simulink library "Ice_Storage"  (R2018b)
settings: Solver=ode45  StartTime=0.0  StopTime=10.0  RelTol=1e-3  EnableMultiTasking=on
undefined symbols (not defined in the file): A_earth, delta_grd, h_ini, U_earth, UA_tank, V_earth, ztilde
libraries: carnot x2
settings Model: Creator=drhf  LastModifiedBy=drhf
settings DataIOCC: LimitDataPoints=on  SaveFormat=Array  SignalLoggingSaveFormat=ModelDataLogs
settings OptimizationCC: ExpressionDepthLimit=2147483647  LifeSpan=inf
settings DebuggingCC: UnderspecifiedInitializationDetection=Classic  MergeDetectMultiDrivingBlocksExec=none  SolverPrmCheckMsg=warning  FcnCallInpInsideContextMsg=warning  StateNameClashWarn=warning  SFUnexpectedBacktrackingDiag=warning  SFNoUnconditionalDefaultTransitionDiag=warning  SFExecutionAtInitializationDiag=none
settings HardwareCC: ProdBitPerPointer=32  ProdBitPerSizeT=32  ProdBitPerPtrDiffT=32  ProdLargestAtomicFloat=None  ProdIntDivRoundTo=Undefined  ProdEndianess=Unspecified  ProdWordSize=32  ProdHWDeviceType=32-bit Generic
settings ModelReferenceCC: PropagateSignalLabelsOutOfModel=off
settings SFSimCC: SimUseLocalCustomCode=off
settings RTWCC: RTWUseLocalCustomCode=off
settings CodeAppCC: StateflowObjectComments=on
settings GRTTargetCC: TargetLangStandard=C89/C90 (ANSI)  GeneratePreprocessorConditionals=Disable all  CombineOutputUpdateFcns=off  GRTInterface=on
settings ConfigComp: CovMetricSettings=dw  CovHtmlReporting=on  CovSaveCumulativeToWorkspaceVar=on  CovSaveSingleToWorkspaceVar=on  CovExternalEMLEnable=off

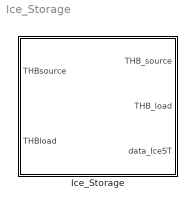
== system Ice_Storage ==
  Ice_Storage : Subsystem  mask(Ice Storage){vol=10, h=2.3, z=3.2, Lhx_sol=195, Ulen_sol=1500/28/9.5            % 1.5 kW at dT = 9.5 K with a 28 m tube of outer diameter 32 mm, mpc_sol=1*3500, Lhx_hp=7*50, Ulen_hp=1500/28/9.5            % 1.5 kW at dT = 9.5 K with a 28 m tube of outer diameter 32 mm, mpc_hp=1*3500, dearth=0.5, cond_ground=2, cp_ground=800, rho_ground=2500, Tmeanoutside=11, deltathetae=9.3, tshift=319, f_ice=0, t_ini=15}
      mask prompts: vol "volume [m³]"; h "water level from bottom in m"; z "depth of baseplate from upper surface [m]"; Lhx_sol "Length in m"; Ulen_sol "Heat transfer per length in W/K/m"; mpc_sol "Thermal capacity per length in J/K/m"; Lhx_hp "Length in m"; Ulen_hp "Heat transfer per length in W/K/m"; mpc_hp "Thermal capacity per length in J/K/m"; dearth "thickness of surrounding earth layer [m]"; cond_ground "conductivity of ground [W/(m*K)]"; cp_ground "capacity of ground [J/(kg*K)]"; rho_ground "density of ground [kg/m^3]"; Tmeanoutside "mean outside temperature over one year [°C]"; deltathetae "amplitude of outside ambient temperatures over one year [°C]"; tshift "time shift where ambient temperature sine-curve shows a minimum [h]"; f_ice "Initial ice fraction, must be in the range (0..1)"; t_ini "Initial temperature in °C, must be >= 0 °C"
      mask help: One node model of an ice storage with a charging (source) and discharging (load) heat exchanger. See help file for a detailed description and the data_IceST output.
      mask init:
      | [h_ini, t_ini, A, B, dt, dw, ztilde, delta_grd, U_earth, A_earth, V_earth, UA_tank] = ...
      |     CarnotCallbacks_IceStorage(f_ice, t_ini, vol, h, z, dearth, cond_ground, rho_ground, cp_ground);
      mask Help: web(fullfile(path_carnot('help'),'ice_storage.html'),'-helpbrowser')
      mask TypeOptions Lhx_sol: Heat_Exchanger_Solar/Lhx
      mask TypeOptions Ulen_sol: Heat_Exchanger_Solar/Ulen
      mask TypeOptions mpc_sol: Heat_Exchanger_Solar/mpc_hp
      mask TypeOptions Lhx_hp: Heat_Exchanger_HP/Lhx
      mask TypeOptions Ulen_hp: Heat_Exchanger_HP/Ulen
      mask TypeOptions mpc_hp: Heat_Exchanger_HP/mpc_hp
      mask DialogControl Container4 Prompt: Ice Storage
      mask DialogControl Container11 Prompt: Source Heat Exchanger Pipe
      mask DialogControl Container8 Prompt: Load Heat Exchanger Pipe
      mask DialogControl Container10 Prompt: Surrounding Ground
      mask DialogControl Container6 Prompt: Initial Values
      mask DialogControl Control2 Prompt: The model is initialized with an ice fraction and a temperature. The temperature is only relevant if the initial ice fraction is 0. For ice fractions above 0 the initial temperature is automatically set to 0 °C.
      mask Display: plot(0,0,100,100,[20,30,40,50,60,70,70,60,50,40,30,20,20],[70,90,84,84,90,70,20,13,10,10,13,20,70],[60,50,40,30],[90,95,95,90],[70,60,50,40,30,20],[70,64,60,60,64,70],[45,45],[20,50],[56,35],[35,35],[53,37],[26,44],[53,37],[44,26],[48,45,42],[46,43,46],[54,51,54],[33,35,38],[48,45,42],[24,28,23],[37,40,37],[32,35,38])

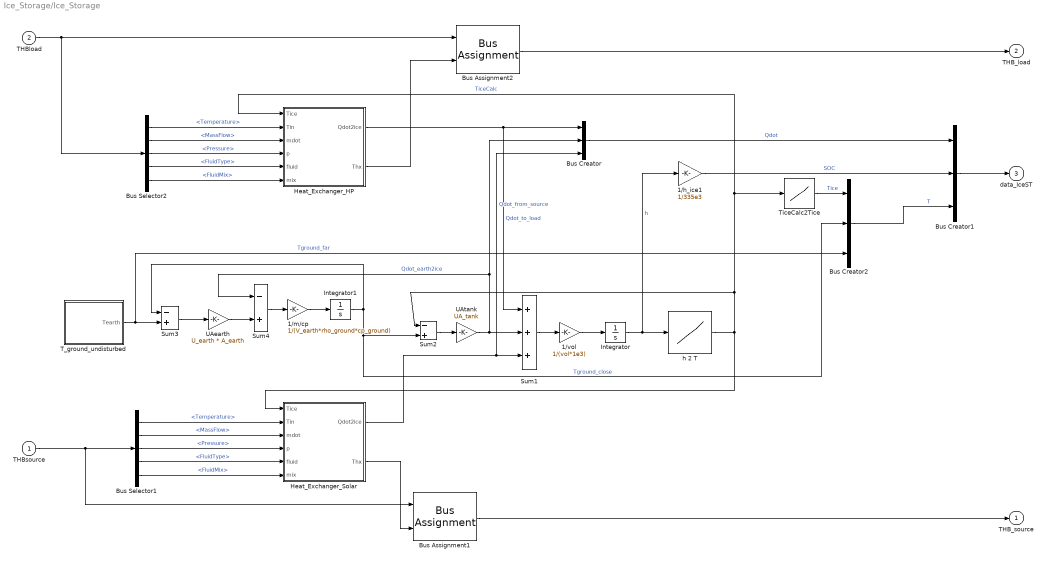
== system Ice_Storage/Ice_Storage ==
  THBsource : Inport
  THBload : Inport  Port=2
  1/h_ice1 : Gain  Gain=1/335e3  SaturateOnIntegerOverflow=on  OutDataTypeStr=Inherit: Same as input  ParamDataTypeStr=Inherit: Same as input
  1/m/cp : Gain  Gain=1/(V_earth*rho_ground*cp_ground)  SaturateOnIntegerOverflow=on  OutDataTypeStr=Inherit: Same as input  ParamDataTypeStr=Inherit: Same as input
  1/vol : Gain  Gain=1/(vol*1e3)  SaturateOnIntegerOverflow=on  OutDataTypeStr=Inherit: Same as input  ParamDataTypeStr=Inherit: Same as input
  Bus Assignment1 : BusAssignment  AssignedSignals=Temperature
  Bus Assignment2 : BusAssignment  AssignedSignals=Temperature
  Bus Creator : BusCreator  Inputs=3
  Bus Creator1 : BusCreator  Inputs=3
  Bus Creator2 : BusCreator  Inputs=3
  Bus Selector1 : BusSelector  OutputSignals=Temperature,MassFlow,Pressure,FluidType,FluidMix
  Bus Selector2 : BusSelector  OutputSignals=Temperature,MassFlow,Pressure,FluidType,FluidMix
  Heat_Exchanger_HP : Subsystem  mask{Lhx=Lhx_hp, Ulen=Ulen_hp, mpc_hp=mpc_hp}
      mask prompts: Lhx "Length of heat exchanger pipe in m"; Ulen "Heat transfer of pipe per length in W/K/m"; mpc_hp "Thermal capacity of pipe per length in J/K/m"
      mask TypeOptions Lhx: Constant/Value
      mask TypeOptions Ulen: U_length/Gain
      mask TypeOptions mpc_hp: Constant1/Value
  Heat_Exchanger_Solar : Subsystem  mask{Lhx=Lhx_sol, Ulen=Ulen_sol, mpc_hp=mpc_sol}
      mask prompts: Lhx "Length of heat exchanger pipe in m"; Ulen "Heat transfer of pipe per length in W/K/m"; mpc_hp "Thermal capacity of pipe per length in J/K/m"
      mask TypeOptions Lhx: Constant/Value
      mask TypeOptions Ulen: U_length/Gain
      mask TypeOptions mpc_hp: Constant1/Value
  Integrator : Integrator  InitialCondition=h_ini
  Integrator1 : Integrator  InitialCondition=4
  Sum1 : Sum  Inputs=+++  SaturateOnIntegerOverflow=on  InputSameDT=on  OutDataTypeStr=Inherit: Same as first input
  Sum2 : Sum  Inputs=-+  SaturateOnIntegerOverflow=on  InputSameDT=on  OutDataTypeStr=Inherit: Same as first input
  Sum3 : Sum  Inputs=-+  SaturateOnIntegerOverflow=on  InputSameDT=on  OutDataTypeStr=Inherit: Same as first input
  Sum4 : Sum  Inputs=-+  SaturateOnIntegerOverflow=on  InputSameDT=on  OutDataTypeStr=Inherit: Same as first input
  T_ground_undisturbed : Subsystem
  TiceCalc2Tice : Lookup  InputValues=[-10 -3 0 10]  Table=[-10 0 0 10]
  UAearth : Gain  Gain=U_earth * A_earth  SaturateOnIntegerOverflow=on  OutDataTypeStr=Inherit: Same as input  ParamDataTypeStr=Inherit: Same as input
  UAtank : Gain  Gain=UA_tank  SaturateOnIntegerOverflow=on  OutDataTypeStr=Inherit: Same as input  ParamDataTypeStr=Inherit: Same as input
  h 2 T : Lookup  InputValues=[-2060*10 -2060*3 335e3 335e3+4182*10]  Table=[-10 -3 0 10]
  THB_source : Outport
  THB_load : Outport  Port=2
  data_IceST : Outport  Port=3
  wires:
  Bus Creator/1 -> Bus Creator1/1  "Qdot"
  Heat_Exchanger_HP/1(Qdot2ice) -> Sum1/1, Bus Creator/1  "Qdot_to_load"
  THBload/1 -> Bus Assignment2/1, Bus Selector2/1
  Heat_Exchanger_Solar/1(Qdot2ice) -> Sum1/3, Bus Creator/3  "Qdot_from_source"
  h 2 T/1 -> Heat_Exchanger_Solar/1(Tice), Sum2/1, Heat_Exchanger_HP/1(Tice), TiceCalc2Tice/1  "TiceCalc"
  Integrator1/1 -> Bus Creator2/2, Sum2/2, Sum3/1  "Tground_close"
  1/m/cp/1 -> Integrator1/1
  Sum4/1 -> 1/m/cp/1
  UAearth/1 -> Sum4/2
  Sum3/1 -> UAearth/1
  Integrator/1 -> h 2 T/1, 1/h_ice1/1  "h"
  UAtank/1 -> Bus Creator/2, Sum4/1, Sum1/2  "Qdot_earth2ice"
  Sum2/1 -> UAtank/1
  Sum1/1 -> 1/vol/1
  1/vol/1 -> Integrator/1
  Heat_Exchanger_Solar/2(Thx) -> Bus Assignment1/2
  THBsource/1 -> Bus Assignment1/1, Bus Selector1/1
  Bus Creator1/1 -> data_IceST/1
  1/h_ice1/1 -> Bus Creator1/2  "SOC"
  T_ground_undisturbed/1(Tearth) -> Sum3/2, Bus Creator2/3  "Tground_far"
  Bus Creator2/1 -> Bus Creator1/3  "T"
  Bus Assignment1/1 -> THB_source/1
  Bus Selector1/1 -> Heat_Exchanger_Solar/2(Tin)  "<Temperature>"
  Bus Selector1/3 -> Heat_Exchanger_Solar/4(p)  "<Pressure>"
  Bus Selector1/5 -> Heat_Exchanger_Solar/6(mix)  "<FluidMix>"
  Bus Selector1/4 -> Heat_Exchanger_Solar/5(fluid)  "<FluidType>"
  Bus Selector1/2 -> Heat_Exchanger_Solar/3(mdot)  "<MassFlow>"
  Bus Selector2/4 -> Heat_Exchanger_HP/5(fluid)  "<FluidType>"
  Bus Selector2/2 -> Heat_Exchanger_HP/3(mdot)  "<MassFlow>"
  Bus Selector2/5 -> Heat_Exchanger_HP/6(mix)  "<FluidMix>"
  Bus Selector2/3 -> Heat_Exchanger_HP/4(p)  "<Pressure>"
  Bus Selector2/1 -> Heat_Exchanger_HP/2(Tin)  "<Temperature>"
  Bus Assignment2/1 -> THB_load/1
  Heat_Exchanger_HP/2(Thx) -> Bus Assignment2/2
  TiceCalc2Tice/1 -> Bus Creator2/1  "Tice"

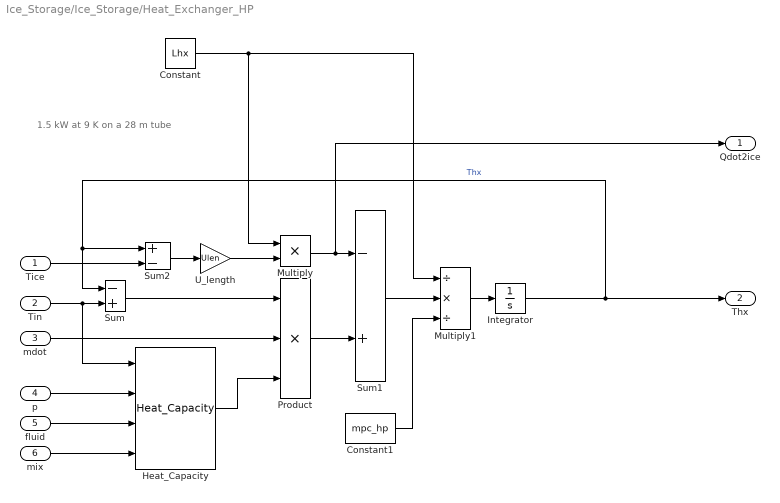
== system Ice_Storage/Ice_Storage/Heat_Exchanger_HP ==
  note: 1.5 kW at 9 K on a 28 m tube
  Tice : Inport
  Tin : Inport  Port=2
  mdot : Inport  Port=3
  p : Inport  Port=4
  fluid : Inport  Port=5
  mix : Inport  Port=6
  Constant : Constant  Value=Lhx
  Constant1 : Constant  Value=mpc_hp
  Heat_Capacity : carnot/Basic/Material_Properties/Heat_Capacity  VariantControl=CarlibClassic  INPUTARGUMENTS=state variables (classic)  DEBUGLEVEL=DEBUGLEVEL  MAXTOTALWARNINGS=inf  MAXCONSECUTIVEWARNINGS=inf  WRITETOFILE=0  FILENAME='errors.txt'
      settings: SourceProductName=Carnot
  Integrator : Integrator  InitialCondition=t_ini
  Multiply : Product
  Multiply1 : Product  Inputs=/*/
  Product : Product  Inputs=3  SaturateOnIntegerOverflow=on  InputSameDT=on  OutDataTypeStr=Inherit: Same as first input
  Sum : Sum  Inputs=-+  SaturateOnIntegerOverflow=on  InputSameDT=on  OutDataTypeStr=Inherit: Same as first input
  Sum1 : Sum  Inputs=-+  SaturateOnIntegerOverflow=on  InputSameDT=on  OutDataTypeStr=Inherit: Same as first input
  Sum2 : Sum  Inputs=+-  SaturateOnIntegerOverflow=on  InputSameDT=on  OutDataTypeStr=Inherit: Same as first input
  U_length : Gain  Gain=Ulen  SaturateOnIntegerOverflow=on  OutDataTypeStr=Inherit: Same as input  ParamDataTypeStr=Inherit: Same as input
  Qdot2ice : Outport
  Thx : Outport  Port=2
  wires:
  Tin/1 -> Heat_Capacity/1, Sum/2
  Integrator/1 -> Sum/1, Sum2/1, Thx/1  "Thx"
  Product/1 -> Sum1/2
  Heat_Capacity/1 -> Product/3
  Sum/1 -> Product/1
  Sum2/1 -> U_length/1
  mdot/1 -> Product/2
  p/1 -> Heat_Capacity/2
  fluid/1 -> Heat_Capacity/3
  mix/1 -> Heat_Capacity/4
  Tice/1 -> Sum2/2
  U_length/1 -> Multiply/2
  Multiply/1 -> Qdot2ice/1, Sum1/1
  Constant/1 -> Multiply1/1, Multiply/1
  Constant1/1 -> Multiply1/3
  Multiply1/1 -> Integrator/1
  Sum1/1 -> Multiply1/2

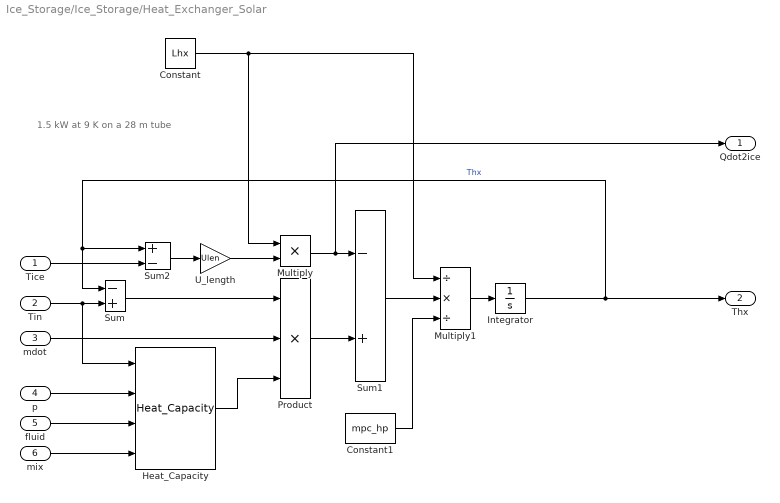
== system Ice_Storage/Ice_Storage/Heat_Exchanger_Solar ==
  note: 1.5 kW at 9 K on a 28 m tube
  Tice : Inport
  Tin : Inport  Port=2
  mdot : Inport  Port=3
  p : Inport  Port=4
  fluid : Inport  Port=5
  mix : Inport  Port=6
  Constant : Constant  Value=Lhx
  Constant1 : Constant  Value=mpc_hp
  Heat_Capacity : carnot/Basic/Material_Properties/Heat_Capacity  VariantControl=CarlibClassic  INPUTARGUMENTS=state variables (classic)  DEBUGLEVEL=DEBUGLEVEL  MAXTOTALWARNINGS=inf  MAXCONSECUTIVEWARNINGS=inf  WRITETOFILE=0  FILENAME='errors.txt'
      settings: SourceProductName=Carnot
  Integrator : Integrator  InitialCondition=t_ini
  Multiply : Product
  Multiply1 : Product  Inputs=/*/
  Product : Product  Inputs=3  SaturateOnIntegerOverflow=on  InputSameDT=on  OutDataTypeStr=Inherit: Same as first input
  Sum : Sum  Inputs=-+  SaturateOnIntegerOverflow=on  InputSameDT=on  OutDataTypeStr=Inherit: Same as first input
  Sum1 : Sum  Inputs=-+  SaturateOnIntegerOverflow=on  InputSameDT=on  OutDataTypeStr=Inherit: Same as first input
  Sum2 : Sum  Inputs=+-  SaturateOnIntegerOverflow=on  InputSameDT=on  OutDataTypeStr=Inherit: Same as first input
  U_length : Gain  Gain=Ulen  SaturateOnIntegerOverflow=on  OutDataTypeStr=Inherit: Same as input  ParamDataTypeStr=Inherit: Same as input
  Qdot2ice : Outport
  Thx : Outport  Port=2
  wires:
  Sum1/1 -> Multiply1/2
  Multiply1/1 -> Integrator/1
  Constant1/1 -> Multiply1/3
  Constant/1 -> Multiply/1, Multiply1/1
  Multiply/1 -> Sum1/1, Qdot2ice/1
  U_length/1 -> Multiply/2
  Tice/1 -> Sum2/2
  mix/1 -> Heat_Capacity/4
  fluid/1 -> Heat_Capacity/3
  p/1 -> Heat_Capacity/2
  mdot/1 -> Product/2
  Sum2/1 -> U_length/1
  Sum/1 -> Product/1
  Heat_Capacity/1 -> Product/3
  Product/1 -> Sum1/2
  Integrator/1 -> Thx/1, Sum2/1, Sum/1  "Thx"
  Tin/1 -> Sum/2, Heat_Capacity/1

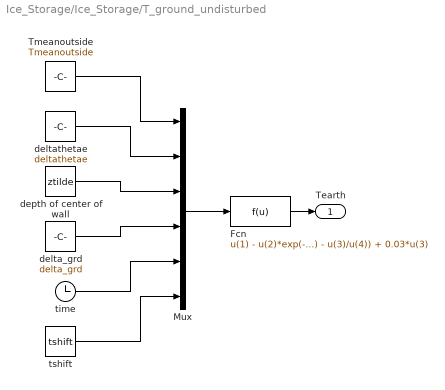
== system Ice_Storage/Ice_Storage/T_ground_undisturbed ==
  Fcn : Fcn  Expr=u(1) - u(2)*exp(-u(3)/u(4))*cos(2*pi*(u(5)-u(6)*3600)/(365*24*3600) - u(3)/u(4)) + 0.03*u(3)
  Mux : Mux  Inputs=6
  Tmeanoutside : Constant  Value=Tmeanoutside
  delta_grd : Constant  Value=delta_grd
  deltathetae : Constant  Value=deltathetae
  depth of center of wall : Constant  Value=ztilde
  time : Clock
  tshift : Constant  Value=tshift
  Tearth : Outport
  wires:
  Fcn/1 -> Tearth/1
  Mux/1 -> Fcn/1
  tshift/1 -> Mux/6
  time/1 -> Mux/5
  delta_grd/1 -> Mux/4
  depth of center of wall/1 -> Mux/3
  deltathetae/1 -> Mux/2
  Tmeanoutside/1 -> Mux/1
